simulink model "real_model"  (R2023a)
settings: Solver=VariableStepAuto  StartTime=0.0  StopTime=3072.3364  RelTol=1e-6  AbsTol=1e-7
undefined symbols (not defined in the file or in its folder): state_dim, state_sens
settings Model: Creator=bryan  LastModifiedBy=bryan

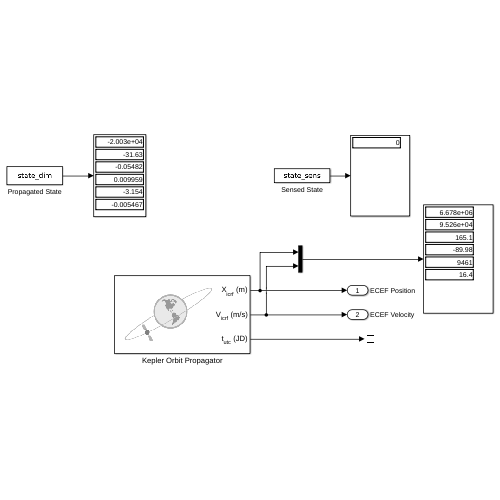
[thumbnail: Simulink's stored preview of the top-level diagram]
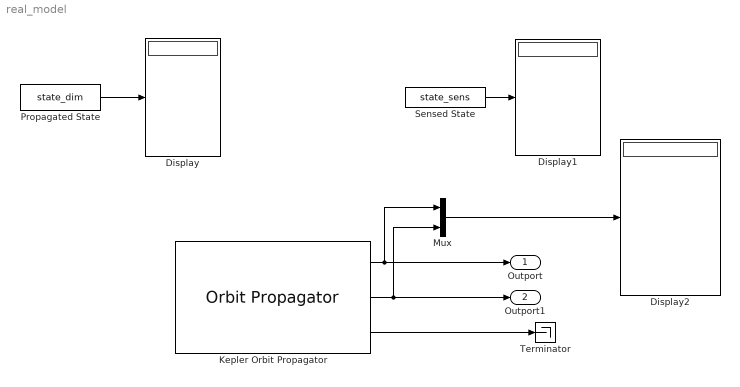
== system real_model ==
  Display : Display
  Display1 : Display
  Display2 : Display
  Kepler Orbit Propagator : OrbitPropagator  outportFrame=Fixed-frame  startDate=2458488  semiMajorAxis=mission.Satellite.SemiMajorAxis  eccentricity=mission.Satellite.Eccentricity  inclination=mission.Satellite.Inclination  raan=mission.Satellite.RAAN  argPeriapsis=mission.Satellite.ArgOfPeriapsis  trueAnomaly=mission.Satellite.TrueAnomaly  inertialPosition=[3649700.0 3308200.0 -4676600.0]  inertialVelocity=[-2750.8 6666.4 2573.4]  fixedPosition=[-4142689.0 -2676864.7 -4669861.6]  fixedVelocity=[1452.7 -6720.7 2568.1]  gravityModel=Point-mass  customR=3396200  customMu=4.305e13  customJ2=1.0826269e-03  customOmega=4.06125949e-3  outputTransform=on
  Mux : Mux  Inputs=2
  Propagated State : Constant  Value=state_dim  VectorParams1D=off
  Sensed State : Constant  Value=state_sens  VectorParams1D=off
  Terminator : Terminator
  Outport : Outport  SignalName=ECEF Position
  Outport1 : Outport  Port=2  SignalName=ECEF Velocity
  wires:
  Kepler Orbit Propagator/3 -> Terminator/1
  Kepler Orbit Propagator/1 -> Mux/1, Outport/1
  Kepler Orbit Propagator/2 -> Mux/2, Outport1/1
  Propagated State/1 -> Display/1
  Sensed State/1 -> Display1/1
  Mux/1 -> Display2/1
